simulink model "L07"  (R2020b)
settings: Solver=FixedStepDiscrete  StartTime=0.0  StopTime=40.0  FixedStep=1  RelTol=1e-3
undefined symbols (not defined in the file): a, b
settings Model: Creator=Nic  LastModifiedBy=Nic

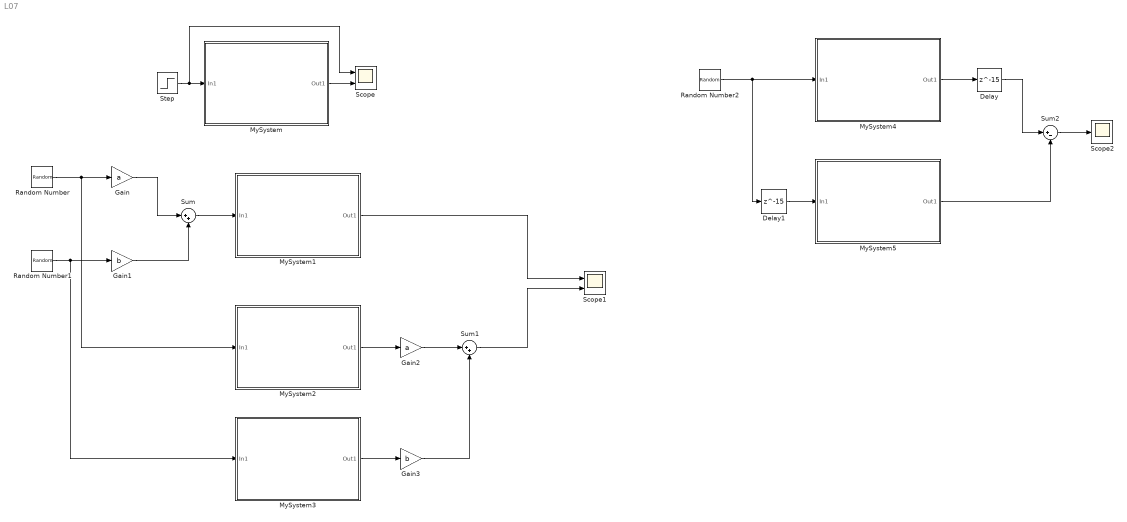
== system L07 ==
  Delay : Delay  DelayLength=15  InitialCondition=0
  Delay1 : Delay  DelayLength=15  InitialCondition=0
  Gain : Gain  Gain=a
  Gain1 : Gain  Gain=b
  Gain2 : Gain  Gain=a
  Gain3 : Gain  Gain=b
  MySystem : Subsystem
  MySystem1 : Subsystem
  MySystem2 : Subsystem
  MySystem3 : Subsystem
  MySystem4 : Subsystem
  MySystem5 : Subsystem
  Random Number : RandomNumber  Seed=12  SampleTime=1
  Random Number1 : RandomNumber  Seed=15  SampleTime=1
  Random Number2 : RandomNumber  Seed=12  SampleTime=1
  Scope : Scope  NumInputPorts=2
  Scope1 : Scope  NumInputPorts=2
  Scope2 : Scope
  Step : Step  SampleTime=0
  Sum : Sum  Inputs=|++
  Sum1 : Sum  Inputs=|++
  Sum2 : Sum  Inputs=|+-
  wires:
  Step/1 -> Scope/1, MySystem/1(In1)
  MySystem/1(Out1) -> Scope/2
  Random Number1/1 -> MySystem3/1(In1), Gain1/1
  Random Number/1 -> MySystem2/1(In1), Gain/1
  Gain/1 -> Sum/1
  Gain1/1 -> Sum/2
  Sum/1 -> MySystem1/1(In1)
  MySystem1/1(Out1) -> Scope1/1
  MySystem2/1(Out1) -> Gain2/1
  MySystem3/1(Out1) -> Gain3/1
  Gain2/1 -> Sum1/1
  Gain3/1 -> Sum1/2
  Sum1/1 -> Scope1/2
  Random Number2/1 -> Delay1/1, MySystem4/1(In1)
  MySystem4/1(Out1) -> Delay/1
  Delay/1 -> Sum2/1
  Delay1/1 -> MySystem5/1(In1)
  MySystem5/1(Out1) -> Sum2/2
  Sum2/1 -> Scope2/1

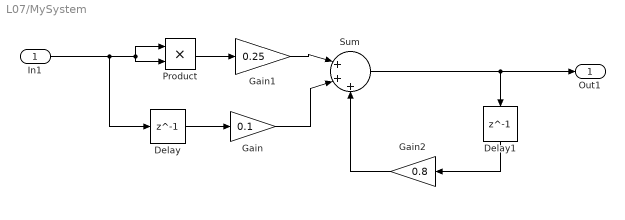
== system L07/MySystem ==
  In1 : Inport
  Delay : Delay  DelayLength=1  InitialCondition=0
  Delay1 : Delay  DelayLength=1  InitialCondition=0
  Gain : Gain  Gain=0.1
  Gain1 : Gain  Gain=0.25
  Gain2 : Gain  Gain=0.8
  Product : Product
  Sum : Sum  Inputs=|+++
  Out1 : Outport
  wires:
  Delay1/1 -> Gain2/1
  Sum/1 -> Out1/1, Delay1/1
  Gain1/1 -> Sum/1
  Gain2/1 -> Sum/3
  Delay/1 -> Gain/1
  Gain/1 -> Sum/2
  Product/1 -> Gain1/1
  In1/1 -> Product/2, Product/1, Delay/1

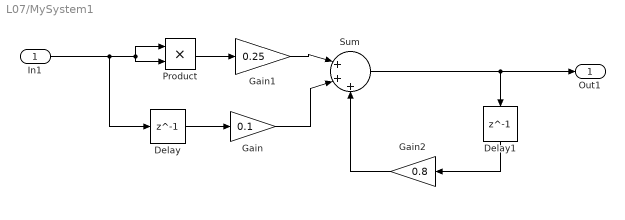
== system L07/MySystem1 ==
  In1 : Inport
  Delay : Delay  DelayLength=1  InitialCondition=0
  Delay1 : Delay  DelayLength=1  InitialCondition=0
  Gain : Gain  Gain=0.1
  Gain1 : Gain  Gain=0.25
  Gain2 : Gain  Gain=0.8
  Product : Product
  Sum : Sum  Inputs=|+++
  Out1 : Outport
  wires:
  Delay1/1 -> Gain2/1
  Sum/1 -> Out1/1, Delay1/1
  Gain1/1 -> Sum/1
  Gain2/1 -> Sum/3
  Delay/1 -> Gain/1
  Gain/1 -> Sum/2
  Product/1 -> Gain1/1
  In1/1 -> Product/2, Product/1, Delay/1

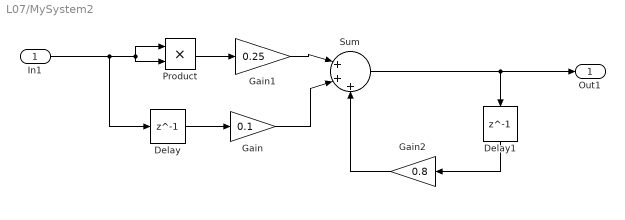
== system L07/MySystem2 ==
  In1 : Inport
  Delay : Delay  DelayLength=1  InitialCondition=0
  Delay1 : Delay  DelayLength=1  InitialCondition=0
  Gain : Gain  Gain=0.1
  Gain1 : Gain  Gain=0.25
  Gain2 : Gain  Gain=0.8
  Product : Product
  Sum : Sum  Inputs=|+++
  Out1 : Outport
  wires:
  Delay1/1 -> Gain2/1
  Sum/1 -> Out1/1, Delay1/1
  Gain1/1 -> Sum/1
  Gain2/1 -> Sum/3
  Delay/1 -> Gain/1
  Gain/1 -> Sum/2
  Product/1 -> Gain1/1
  In1/1 -> Product/2, Product/1, Delay/1

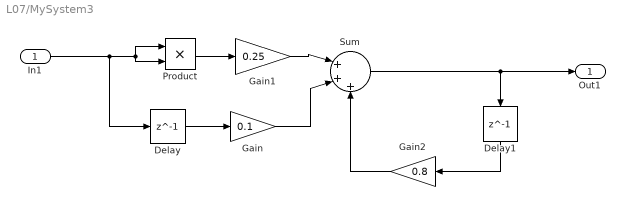
== system L07/MySystem3 ==
  In1 : Inport
  Delay : Delay  DelayLength=1  InitialCondition=0
  Delay1 : Delay  DelayLength=1  InitialCondition=0
  Gain : Gain  Gain=0.1
  Gain1 : Gain  Gain=0.25
  Gain2 : Gain  Gain=0.8
  Product : Product
  Sum : Sum  Inputs=|+++
  Out1 : Outport
  wires:
  Delay1/1 -> Gain2/1
  Sum/1 -> Out1/1, Delay1/1
  Gain1/1 -> Sum/1
  Gain2/1 -> Sum/3
  Delay/1 -> Gain/1
  Gain/1 -> Sum/2
  Product/1 -> Gain1/1
  In1/1 -> Product/2, Product/1, Delay/1

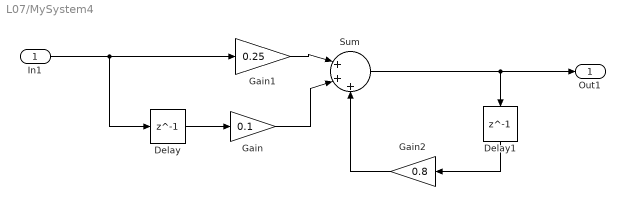
== system L07/MySystem4 ==
  In1 : Inport
  Delay : Delay  DelayLength=1  InitialCondition=0
  Delay1 : Delay  DelayLength=1  InitialCondition=0
  Gain : Gain  Gain=0.1
  Gain1 : Gain  Gain=0.25
  Gain2 : Gain  Gain=0.8
  Sum : Sum  Inputs=|+++
  Out1 : Outport
  wires:
  Delay1/1 -> Gain2/1
  Sum/1 -> Out1/1, Delay1/1
  Gain1/1 -> Sum/1
  Gain2/1 -> Sum/3
  Delay/1 -> Gain/1
  Gain/1 -> Sum/2
  In1/1 -> Gain1/1, Delay/1

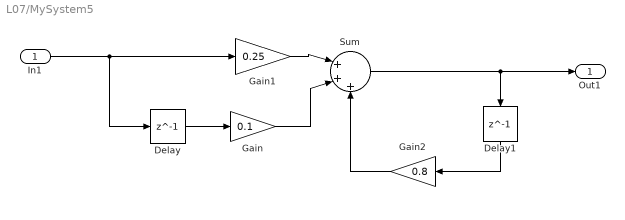
== system L07/MySystem5 ==
  In1 : Inport
  Delay : Delay  DelayLength=1  InitialCondition=0
  Delay1 : Delay  DelayLength=1  InitialCondition=0
  Gain : Gain  Gain=0.1
  Gain1 : Gain  Gain=0.25
  Gain2 : Gain  Gain=0.8
  Sum : Sum  Inputs=|+++
  Out1 : Outport
  wires:
  In1/1 -> Delay/1, Gain1/1
  Gain/1 -> Sum/2
  Delay/1 -> Gain/1
  Gain2/1 -> Sum/3
  Gain1/1 -> Sum/1
  Sum/1 -> Delay1/1, Out1/1
  Delay1/1 -> Gain2/1
